simulink model "Communication"  (R2024b)
settings: Solver=FixedStepDiscrete  StartTime=0.0  StopTime=Inf  FixedStep=Ts  RelTol=1e-3  EnableMultiTasking=on
model workspace (MATLAB code in the model file):
  | %example
  | Vdc = 300 ; % V
  | Trated = 0.8 ; % N.m
  | Tmax = 1.2 ; % N.m
  | Rs = 18.7 ; % Ohm
  | L = 0.02682 ; % H
  | Jm = 2.26e-5 ; % Kg.m^2
  | P = 2 ; % number of pole pairs
  | B = 1.349e-5 ; % N.m/(rad/s)
  | lamda = 0.1716 ; % Wb
  | T=(1/10000) ; % Switching period (s)
  | Ts=10e-6 ; % Sampling time of the solver
  | 
  | gama=0.95;
  | zeta_current=0.9;
  | zeta_speed=0.9;
  | %current controller
  | b_iq=1/L;
  | b_id=1/L;
  | a_id=Rs/L;
  | a_iq=Rs/L;
  | Wn_d=(a_id/(1-gama));
  | Wn_q=(a_iq/(1-gama));
  | Ki_id=(Wn_d^2)/b_id;
  | Ki_iq=(Wn_q^2)/b_iq;
  | Kp_id=((2*zeta_current*Wn_d)-(a_id))/b_id;
  | Kp_iq=((2*zeta_current*Wn_q)-(a_iq))/b_iq;
  | 
  | %Speed controller
  | a_speed=B/Jm;
  | b_speed=(1)/Jm;
  | Wn_speed=Wn_q/10;
  | Ki_speed=(Wn_speed^2)/b_speed;
  | Kp_speed=(((2*zeta_speed*Wn_speed)-(a_speed))/b_speed);
  | 
  | %System Limitations
  | Max_Speed=4100; %RPM
  | Wbase_mech=3100;%RPM
  | Pmax=Wbase_mech*(pi/30)*Trated; %Watt
  | 
  | 
  | %Set points
  | Ref_Speed=3000;%RPM
undefined symbols (not defined in the file): C28x, CPU1, CPU2
libraries: c2837xDlib x1, c280xlib x1
settings Model: ExtModeTrigDuration=8  Creator=shefo  LastModifiedBy=ahmed
settings SolverCC: AlgebraicLoopSolver=TrustRegion
settings OptimizationCC: DefaultUnderspecifiedDataType=single  EnhancedBackFolding=on  PassReuseOutputArgsAs=Individual arguments  MaxStackSize=1024  OptimizeBlockOrder=speed  DifferentSizesBufferReuse=on  OptimizationCustomize=off  DenormalBehavior=FlushToZero  EfficientTunableParamExpr=on
settings DebuggingCC: ParameterTunabilityLossMsg=error  UnconnectedInputMsg=warning  UnconnectedOutputMsg=warning  UnconnectedLineMsg=warning
settings HardwareCC: ProdBitPerChar=16  ProdBitPerInt=16  ProdBitPerPointer=32  ProdBitPerSizeT=32  ProdBitPerPtrDiffT=32  ProdLargestAtomicInteger=Integer  ProdLargestAtomicFloat=None  ProdWordSize=16  ProdLongLongMode=on  ProdHWDeviceType=Texas Instruments->C2000
settings ModelReferenceCC: EnableRefExpFcnMdlSchedulingChecks=on
settings SFSimCC: MATLABDynamicMemAlloc=off
settings RTWCC: Description=Embedded Coder  SystemTargetFile=ert.tlc  HardwareBoard=TI Delfino F28379D LaunchPad  TemplateMakefile=ert_default_tmf  Toolchain=Texas Instruments Code Composer Studio (C2000)  GPUComputeCapability=3.5  DLArmComputeVersion=19.05
settings CodeAppCC: ForceParamTrailComments=on  IgnoreCustomStorageClasses=off  OperatorAnnotations=on  SimulinkDataObjDesc=on  SFDataObjDesc=on  InsertBlockDesc=on
settings ERTTargetCC: TargetLangStandard=C99 (ISO)  CodeReplacementLibrary=TI C28x  ExtModeTransport=3  ExtModeStaticAllocSize=10000  InlinedParameterPlacement=Hierarchical  DynamicArrayContainerType=coder::array

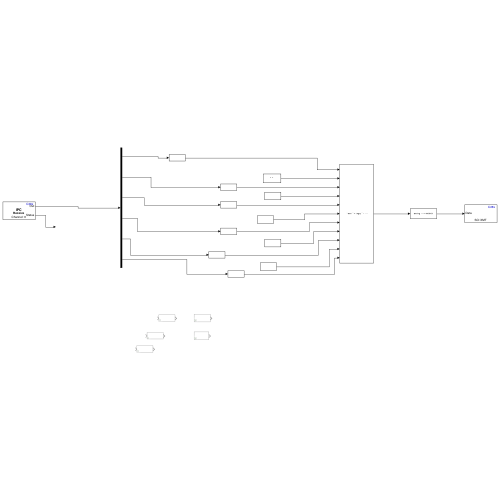
[thumbnail: Simulink's stored preview of the top-level diagram]
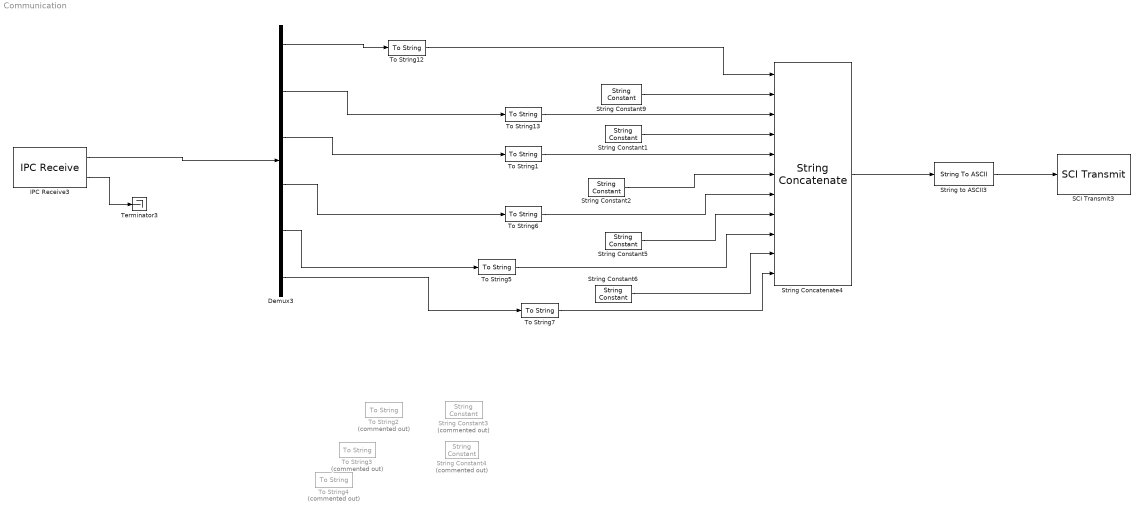
== system Communication ==
  Demux3 : Demux  Outputs=6
  IPC Receive3 : c2837xDlib/IPC Receive  blkParamProc=F2837x  SelectSource=C28x (CPU1/CPU2)  SelectChannel=0  DataType=single  DataLength=6  EnableBlocking=off  SampleTime=1e-4
  SCI Transmit3 : c280xlib/SCI Transmit  sciModule=A  dataHead=''  dataTail="\"\\n\""  frameSize=1  blockingMode=on  outputStatus=off
  String Concatenate4 : StringConcatenate  Inputs=11
  String Constant{1..2,5..6,9} (5 alike) : StringConstant  String="\",\""
  String Constant3 : StringConstant  Commented=on  String="\",\""
  String Constant4 : StringConstant  Commented=on  String="\",\""
  String to ASCII3 : StringToASCII  OutputVectorSize=34
  Terminator3 : Terminator
  To String{1,5..7,12..13} (6 alike) : ToString
  To String2 : ToString  Commented=on
  To String3 : ToString  Commented=on
  To String4 : ToString  Commented=on
  wires:
  IPC Receive3/1 -> Demux3/1
  IPC Receive3/2 -> Terminator3/1
  Demux3/1 -> To String12/1
  Demux3/3 -> To String1/1
  String to ASCII3/1 -> SCI Transmit3/1
  Demux3/2 -> To String13/1
  To String12/1 -> String Concatenate4/1
  String Constant9/1 -> String Concatenate4/2
  To String13/1 -> String Concatenate4/3
  String Constant1/1 -> String Concatenate4/4
  String Concatenate4/1 -> String to ASCII3/1
  To String1/1 -> String Concatenate4/5
  Demux3/4 -> To String6/1
  Demux3/5 -> To String5/1
  String Constant2/1 -> String Concatenate4/6
  To String6/1 -> String Concatenate4/7
  String Constant5/1 -> String Concatenate4/8
  To String5/1 -> String Concatenate4/9
  String Constant6/1 -> String Concatenate4/10
  To String7/1 -> String Concatenate4/11
  Demux3/6 -> To String7/1
